simulink model "Task3"  (R2019b)
settings: Solver=VariableStepAuto  StartTime=0.0  StopTime=10.0  RelTol=1e-3
settings Model: Creator=12393  LastModifiedBy=12393

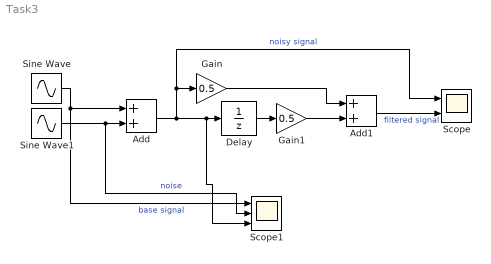
== system Task3 ==
  Add : Sum
  Add1 : Sum
  Delay : UnitDelay  SampleTime=.2  HasFrameUpgradeWarning=on
  Gain : Gain  Gain=0.5
  Gain1 : Gain  Gain=0.5
  Scope : Scope  NumInputPorts=2
  Scope1 : Scope  NumInputPorts=3
  Sine Wave : Sin  Amplitude=10  SampleTime=.2
  Sine Wave1 : Sin  Amplitude=2.5  Frequency=18  SampleTime=.2
  wires:
  Delay/1 -> Gain1/1
  Gain1/1 -> Add1/2
  Gain/1 -> Add1/1
  Add/1 -> Scope1/3, Delay/1, Scope/1, Gain/1  "noisy signal"
  Sine Wave/1 -> Scope1/1, Add/1  "base signal"
  Sine Wave1/1 -> Scope1/2, Add/2  "noise"
  Add1/1 -> Scope/2  "filtered signal"
